simulink model "Vertical_model"  (R2025b)
settings: Solver=ode4  StartTime=0.0  StopTime=simu.t_end  RelTol=1e-3
values from neighbouring files (symbols this model uses):
  cs = 3000    [main_FRF.m]    (also in main_vertical.m = 5000)
  ct = tir.cz    [main_FRF.m]    (also in main_vertical.m)
  ks = susp.kF    [main_FRF.m]    (also in main_vertical.m)
  kt = tir.kz    [main_FRF.m]    (also in main_vertical.m)
  ms = m*lR/l/2 - mu    [main_FRF.m]    (also in main_vertical.m = m * lR / l - mu; quarter_car_model.m = 320)
  mu = susp.muF    [main_FRF.m]    (also in main_vertical.m; quarter_car_model.m = 45)
undefined symbols (not defined in the file or in its folder): ctrl, road, simu
settings Model: Creator=babys  LastModifiedBy=babys

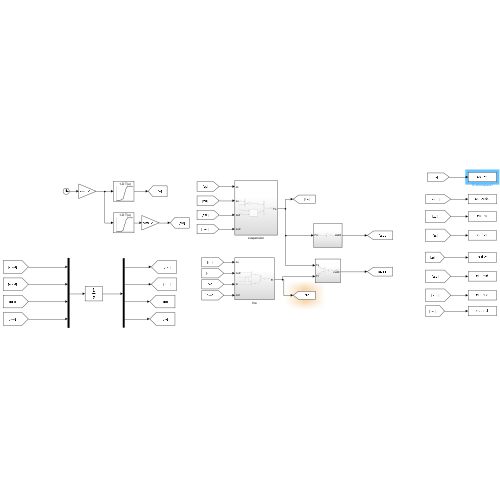
[thumbnail: Simulink's stored preview of the top-level diagram]
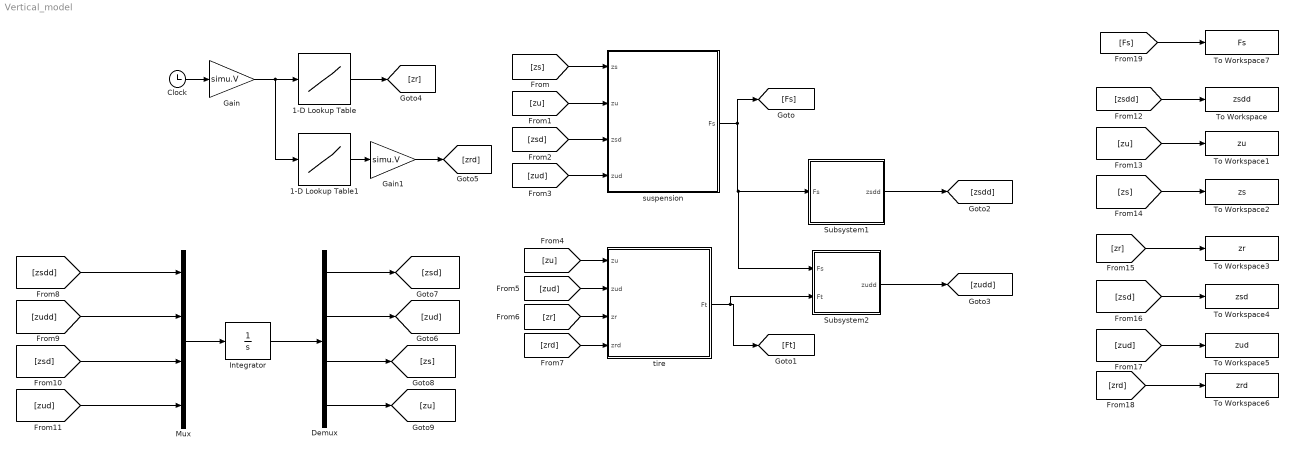
== system Vertical_model ==
  1-D Lookup Table : Lookup_n-D  NumberOfTableDimensions=1  BreakpointsForDimension1=road.s  Table=road.z  InternalRulePriority=Speed  RndMeth=Simplest
  1-D Lookup Table1 : Lookup_n-D  NumberOfTableDimensions=1  BreakpointsForDimension1=road.s  Table=road.z1  InternalRulePriority=Speed  RndMeth=Simplest
  Clock : Clock
  Demux : Demux
  Gain : Gain  Gain=simu.V
  Gain1 : Gain  Gain=simu.V
  Integrator : Integrator  InitialCondition=simu.IC
  Mux : Mux
  Subsystem1 : Subsystem
  Subsystem2 : Subsystem
  To Workspace : ToWorkspace  VariableName=zsdd  SaveFormat=Timeseries  SampleTime=-1
  To Workspace1 : ToWorkspace  VariableName=zu  SaveFormat=Timeseries  SampleTime=-1
  To Workspace2 : ToWorkspace  VariableName=zs  SaveFormat=Timeseries  SampleTime=-1
  To Workspace3 : ToWorkspace  VariableName=zr  SaveFormat=Timeseries  SampleTime=-1
  To Workspace4 : ToWorkspace  VariableName=zsd  SaveFormat=Timeseries  SampleTime=-1
  To Workspace5 : ToWorkspace  VariableName=zud  SaveFormat=Timeseries  SampleTime=-1
  To Workspace6 : ToWorkspace  VariableName=zrd  SaveFormat=Timeseries  SampleTime=-1
  To Workspace7 : ToWorkspace  VariableName=Fs  SaveFormat=Timeseries  SampleTime=-1
  suspension : Subsystem
  tire : Subsystem
  wires:
  [zs] -> suspension/1(zs)
  [zu] -> suspension/2(zu)
  [zsd] -> suspension/3(zsd)
  [zud] -> suspension/4(zud)
  suspension/1(Fs) -> Subsystem2/1(Fs), Subsystem1/1(Fs), [Fs]
  [zu] -> tire/1(zu)
  [zud] -> tire/2(zud)
  [zr] -> tire/3(zr)
  [zrd] -> tire/4(zrd)
  tire/1(Ft) -> Subsystem2/2(Ft), [Ft]
  Subsystem1/1(zsdd) -> [zsdd]
  Subsystem2/1(zudd) -> [zudd]
  Clock/1 -> Gain/1
  Gain/1 -> 1-D Lookup Table1/1, 1-D Lookup Table/1
  1-D Lookup Table/1 -> [zr]
  1-D Lookup Table1/1 -> Gain1/1
  Gain1/1 -> [zrd]
  Integrator/1 -> Demux/1
  Mux/1 -> Integrator/1
  [zsdd] -> Mux/1
  [zudd] -> Mux/2
  [zsd] -> Mux/3
  [zud] -> Mux/4
  Demux/2 -> [zud]
  Demux/1 -> [zsd]
  Demux/3 -> [zs]
  Demux/4 -> [zu]
  [zsdd] -> To Workspace/1
  [zu] -> To Workspace1/1
  [zs] -> To Workspace2/1
  [zr] -> To Workspace3/1
  [zsd] -> To Workspace4/1
  [zud] -> To Workspace5/1
  [zrd] -> To Workspace6/1
  [Fs] -> To Workspace7/1

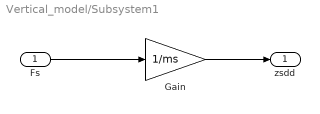
== system Vertical_model/Subsystem1 ==
  Fs : Inport
  Gain : Gain  Gain=1/ms
  zsdd : Outport
  wires:
  Fs/1 -> Gain/1
  Gain/1 -> zsdd/1

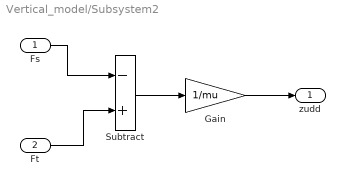
== system Vertical_model/Subsystem2 ==
  Fs : Inport
  Ft : Inport  Port=2
  Gain : Gain  Gain=1/mu
  Subtract : Sum  Inputs=-+
  zudd : Outport
  wires:
  Ft/1 -> Subtract/2
  Fs/1 -> Subtract/1
  Subtract/1 -> Gain/1
  Gain/1 -> zudd/1

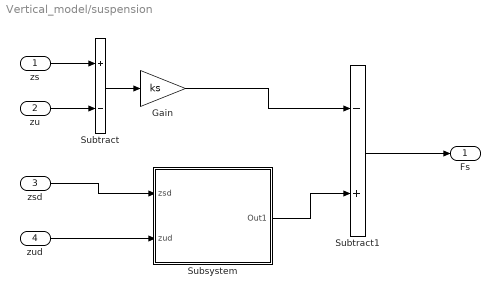
== system Vertical_model/suspension ==
  zs : Inport
  zu : Inport  Port=2
  zsd : Inport  Port=3
  zud : Inport  Port=4
  Gain : Gain  Gain=ks
  Subsystem : Subsystem
  Subtract : Sum  Inputs=+-
  Subtract1 : Sum  Inputs=-+
  Fs : Outport
  wires:
  zs/1 -> Subtract/1
  zu/1 -> Subtract/2
  Subtract/1 -> Gain/1
  zsd/1 -> Subsystem/1(zsd)
  zud/1 -> Subsystem/2(zud)
  Subsystem/1(Out1) -> Subtract1/2
  Gain/1 -> Subtract1/1
  Subtract1/1 -> Fs/1

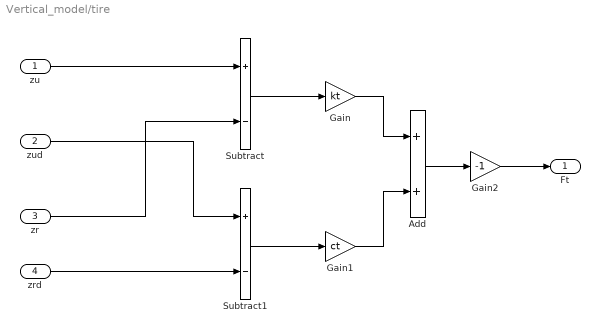
== system Vertical_model/tire ==
  zu : Inport
  zud : Inport  Port=2
  zr : Inport  Port=3
  zrd : Inport  Port=4
  Add : Sum
  Gain : Gain  Gain=kt
  Gain1 : Gain  Gain=ct
  Gain2 : Gain  Gain=-1
  Subtract : Sum  Inputs=+-
  Subtract1 : Sum  Inputs=+-
  Ft : Outport
  wires:
  zu/1 -> Subtract/1
  zr/1 -> Subtract/2
  zud/1 -> Subtract1/1
  zrd/1 -> Subtract1/2
  Subtract/1 -> Gain/1
  Subtract1/1 -> Gain1/1
  Gain/1 -> Add/1
  Gain1/1 -> Add/2
  Add/1 -> Gain2/1
  Gain2/1 -> Ft/1

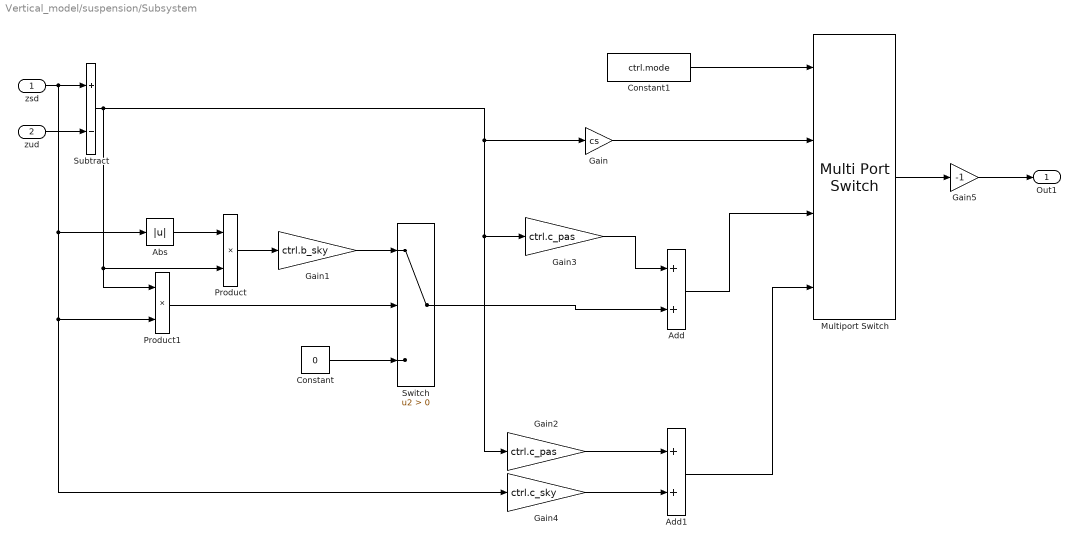
== system Vertical_model/suspension/Subsystem ==
  zsd : Inport
  zud : Inport  Port=2
  Abs : Abs  SaturateOnIntegerOverflow=off
  Add : Sum
  Add1 : Sum
  Constant : Constant  Value=0
  Constant1 : Constant  Value=ctrl.mode
  Gain : Gain  Gain=cs
  Gain1 : Gain  Gain=ctrl.b_sky
  Gain2 : Gain  Gain=ctrl.c_pas
  Gain3 : Gain  Gain=ctrl.c_pas
  Gain4 : Gain  Gain=ctrl.c_sky
  Gain5 : Gain  Gain=-1
  Multiport Switch : MultiPortSwitch  DataPortOrder=Zero-based contiguous  zeroidx=on  SaturateOnIntegerOverflow=off  InputSameDT=off
  Product : Product
  Product1 : Product
  Subtract : Sum  Inputs=+-
  Switch : Switch  Criteria=u2 > Threshold  SaturateOnIntegerOverflow=off  InputSameDT=off
  Out1 : Outport
  wires:
  zsd/1 -> Gain4/1, Product1/2, Abs/1, Subtract/1
  zud/1 -> Subtract/2
  Subtract/1 -> Gain3/1, Gain2/1, Gain/1, Product1/1, Product/2
  Abs/1 -> Product/1
  Product/1 -> Gain1/1
  Gain1/1 -> Switch/1
  Product1/1 -> Switch/2
  Constant/1 -> Switch/3
  Switch/1 -> Add/2
  Gain3/1 -> Add/1
  Gain2/1 -> Add1/1
  Gain4/1 -> Add1/2
  Gain/1 -> Multiport Switch/2
  Add/1 -> Multiport Switch/3
  Add1/1 -> Multiport Switch/4
  Constant1/1 -> Multiport Switch/1
  Gain5/1 -> Out1/1
  Multiport Switch/1 -> Gain5/1
